simulink model "Ex_LinearModel_sml"  (R2018b)
settings: Solver=VariableStepAuto  StartTime=0.0  StopTime=10.0  RelTol=1e-3
settings Model: Creator=user  LastModifiedBy=user

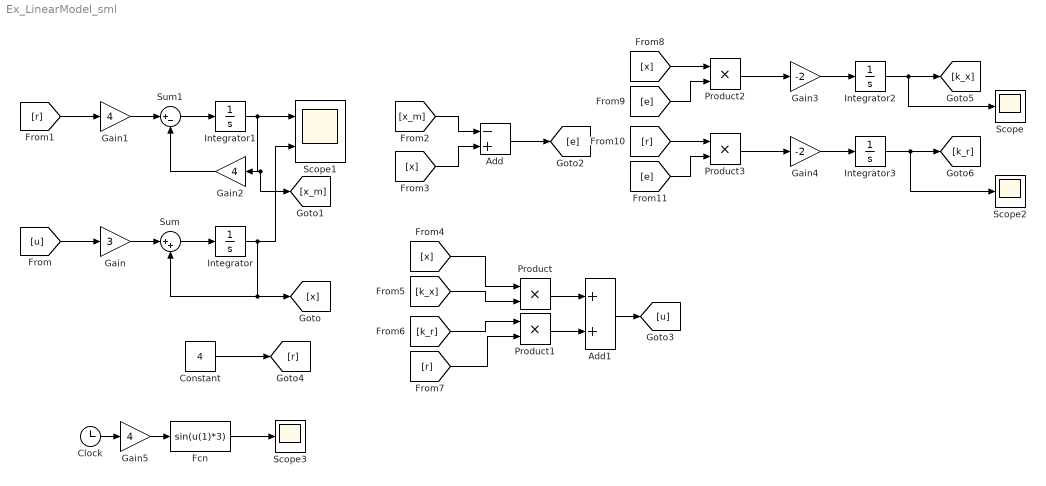
== system Ex_LinearModel_sml ==
  Add : Sum  Inputs=-+
  Add1 : Sum
  Clock : Clock
  Constant : Constant  Value=4
  Fcn : Fcn  Expr=sin(u(1)*3)
  Gain : Gain  Gain=3
  Gain1 : Gain  Gain=4
  Gain2 : Gain  Gain=4
  Gain3 : Gain  Gain=-2
  Gain4 : Gain  Gain=-2
  Gain5 : Gain  Gain=4
  Integrator{,1..3} (4 alike) : Integrator
  Product{,1..3} (4 alike) : Product
  Scope : Scope
  Scope1 : Scope  NumInputPorts=2
  Scope2 : Scope
  Scope3 : Scope
  Sum : Sum  Inputs=|++
  Sum1 : Sum  Inputs=|+-
  wires:
  Sum/1 -> Integrator/1
  Integrator/1 -> Scope1/2, [x], Sum/2
  Gain/1 -> Sum/1
  [u] -> Gain/1
  [r] -> Gain1/1
  Gain1/1 -> Sum1/1
  Integrator1/1 -> Gain2/1, [x_m], Scope1/1
  Sum1/1 -> Integrator1/1
  Gain2/1 -> Sum1/2
  Add/1 -> [e]
  [x] -> Add/2
  [x_m] -> Add/1
  Add1/1 -> [u]
  Product/1 -> Add1/1
  Product1/1 -> Add1/2
  [x] -> Product/1
  [k_x] -> Product/2
  [k_r] -> Product1/1
  [r] -> Product1/2
  Constant/1 -> [r]
  Integrator2/1 -> Scope/1, [k_x]
  [x] -> Product2/1
  Product2/1 -> Gain3/1
  Gain3/1 -> Integrator2/1
  [e] -> Product2/2
  [e] -> Product3/2
  Gain4/1 -> Integrator3/1
  Product3/1 -> Gain4/1
  [r] -> Product3/1
  Integrator3/1 -> Scope2/1, [k_r]
  Clock/1 -> Gain5/1
  Gain5/1 -> Fcn/1
  Fcn/1 -> Scope3/1
